simulink library "statesFileSimulinkLib"  (R2019a)
settings: Solver=VariableStepAuto  StartTime=0.0  StopTime=10.0  RelTol=1e-3
settings Model: Creator=agmotes  LastModifiedBy=agmotes

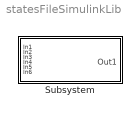
== system statesFileSimulinkLib ==
  Subsystem : Subsystem

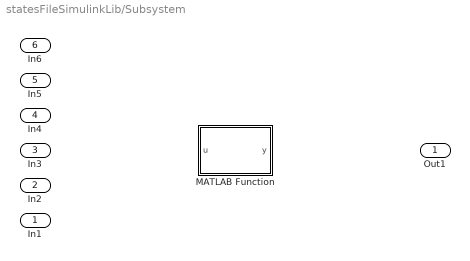
== system statesFileSimulinkLib/Subsystem ==
  In1 : Inport
  In2 : Inport  Port=2
  In3 : Inport  Port=3
  In4 : Inport  Port=4
  In5 : Inport  Port=5
  In6 : Inport  Port=6
  MATLAB Function : MATLAB Function  TreatAsAtomicUnit=on
  Out1 : Outport

== matlab function statesFileSimulinkLib/Subsystem/MATLAB Function ==
  data: u input; y output
function y = fcn(u)

y = u;
